simulink model "autosar_component"  (R2022b)
settings: Solver=FixedStepDiscrete  StartTime=0.0  StopTime=10.0  RelTol=1e-3
PreLoadFcn:
  | PressureEstimation = Simulink.LookupTable;
  | PressureEstimation.Table.DataType = 'auto';
  | PressureEstimation.Table.Min = -1;
  | PressureEstimation.Table.Max = 100;
  | PressureEstimation.Table.Unit = '';
  | PressureEstimation.Table.FieldName = 'Table';
  | PressureEstimation.Table.Description = ...
  |   'Pressure estimation Table data description';
  | PressureEstimation.Table.Value = ...
  |   [0.806253176323533 0.87757598601382 0.957740646602364 0.985153049483995 ...
  |    0.993888908359001 0.997089947885844 0.998445305205399 0.999091830797014 ...
  |    0.999430938454035 0.999622818995239 0.999738270814208 0.999845542107005 ...
  |    0.999937181505709 0.999967346454435 0.999979873928593 0.999985850596962 ...
  |    0.999988872471833;
  |    0.553142316928701 0.687048893636338 0.884928073705099 0.959498363205152 ...
  |    0.983356257320681 0.992081090207251 0.995771008698205 0.997530140187631 ...
  |    0.998452542678774 0.998974388477469 0.99928834538053 0.999580035742161 ...
  |    0.999829204284437 0.999911219910389 0.999945280453193 0.999961530125998 ...
  |    0.999969746130731;
  |    0.37151500208954 0.482612303368962 0.772510257347488 0.91782922063029 ...
  |    0.966202131946129 0.983928124711611 0.991420178702962 0.994990142355732 ...
  |    0.996861498829361 0.997920027607395 0.998556801019289 0.999148366829447 ...
  |    0.999653659903192 0.999819973435009 0.999889041260296 0.999921992055277 ...
  |    0.999938652267344;
  |    0.277667903102846 0.354224278507773 0.634596441906303 0.858155181125974 ...
  |    0.941196863973347 0.972020092047905 0.985064576930091 0.991280051853728 ...
  |    0.994537692220384 0.996380159664924 0.997488437655209 0.998517971150347 ...
  |    0.999397308920136 0.999686725882367 0.999806915357152 0.999864254875951 ...
  |    0.999893246159778;
  |    0.220198954206677 0.278413460665919 0.499509252438175 0.780915653069415 ...
  |    0.90725506963059 0.955734788592824 0.976359298715029 0.986196279487014 ...
  |    0.991353075497716 0.994269777477944 0.996024221776188 0.997653989166547 ...
  |    0.999045967737845 0.999504103593618 0.999694357753908 0.999785123212449 ...
  |    0.99983101483727;
  |    0.181288665766343 0.227999583948868 0.398952953853525 0.690639436957016 ...
  |    0.863705911066113 0.934478804869502 0.964951264217872 0.979525847256624 ...
  |    0.987172517967595 0.991498792106339 0.994101447273549 0.996519319760225 ...
  |    0.998584517171801 0.999264242683749 0.999546520327838 0.999681188248569 ...
  |    0.999749277343391;
  |    0.153200000488606 0.191995727776301 0.330914655151405 0.595646844312617 ...
  |    0.810666723282258 0.90775046318795 0.950492505538488 0.971050093756693 ...
  |    0.981855086965011 0.987972552524888 0.991653973147472 0.995074698970308 ...
  |    0.997996914902605 0.998958792355415 0.999358253074229 0.999548828343865 ...
  |    0.999645185116666;
  |    0.11543102087155 0.144034515174401 0.243979118856238 0.429790108547636 ...
  |    0.682438642375562 0.836880642957011 0.91118032843611 0.947813899384122 ...
  |    0.96722856464052 0.978257580098748 0.984905309066455 0.991088428442116 ...
  |    0.996374579118731 0.998115314543176 0.998838330528732 0.999183288382611 ...
  |    0.999357707498247;
  |    0.0913067476324093 0.113642314330893 0.190658230936961 0.32878428638692 ...
  |    0.545074467052933 0.74462409246358 0.856657795837454 0.91488350746312 ...
  |    0.946318097747896 0.964311517705744 0.975196237184309 0.985342971016168 ...
  |    0.994032962585561 0.996897338116608 0.998087432486324 0.998655313115969 ...
  |    0.998942465702029;
  |    0.074651918860657 0.0927600764089701 0.154689629202074 0.263508735453851 ...
  |    0.428509373032026 0.639187152983657 0.787142203938478 0.87114532382285 ...
  |    0.918076257202549 0.945327888127594 0.961925625193849 0.977463094595001 ...
  |    0.990813081836746 0.995221210749437 0.997053747988697 0.997928394076558 ...
  |    0.998370715394031;
  |    0.0625231108323717 0.0776005353603968 0.128882197432187 0.217821230748895 ...
  |    0.34926567049653 0.533026414797681 0.705799478369783 0.816462064121936 ...
  |    0.881751459546042 0.920583784269911 0.944507657720157 0.967061575702449 ...
  |    0.986544638100701 0.992996396514112 0.995680976286613 0.996962784812372 ...
  |    0.997611133655427;
  |    0.0533383634276856 0.0661461394956957 0.109538590799923 0.18412267971606 ...
  |    0.29255219843447 0.440754788055134 0.618550870186323 0.752132326009762 ...
  |    0.837127815711564 0.889546778841832 0.922421304962653 0.953755223844687 ...
  |    0.981048433857061 0.990126104885857 0.993908561852908 0.995715616100314 ...
  |    0.996629889941259;
  |    0.0461719046290558 0.057223327839534 0.0945575552493262 0.158314103258091 ...
  |    0.249955267698337 0.372825322079962 0.53225525753417 0.681013721820078 ...
  |    0.784760241136601 0.852005161999648 0.895275306545621 0.937186788001516 ...
  |    0.974139712119363 0.986508158488532 0.991672018103867 0.994141054504847 ...
  |    0.995390743685847;
  |    0.0357830207157614 0.0443099388567923 0.0730034651165902 0.121584753293742 ...
  |    0.190411497153518 0.280611299170444 0.394398141965505 0.534281588633688 ...
  |    0.663365830090947 0.758897279500008 0.825346008939808 0.893138430722029 ...
  |    0.955345741069894 0.976600929210005 0.985531654326322 0.989812926442846 ...
  |    0.991982548835214;
  |    0.0286869137234658 0.0355034233512583 0.0583848257268498 0.0969201999867393 ...
  |    0.15104654695125 0.221078862790289 0.307794324372102 0.412602365520382 ...
  |    0.536233487336572 0.649402710410808 0.736919712291059 0.833757084996449 ...
  |    0.928773563241251 0.962402265836581 0.976685081430694 0.98356210634634 ...
  |    0.987054369021;
  |    0.0235863306154347 0.0291800197474993 0.047925624770081 0.0793847279015545 ...
  |    0.123326119357344 0.179727354097858 0.248796241080163 0.331018364047279 ...
  |    0.42724438204184 0.537134400774559 0.637336655478509 0.760335336541618 ...
  |    0.893359883114823 0.943066221776258 0.964537074160009 0.97494574259801 ...
  |    0.980248325729017;
  |    0.0197778405659999 0.0244618918010893 0.0401408494783853 0.0663889743999435 ...
  |    0.1029118379984 0.149540216925307 0.206232624555673 0.273087421642731 ...
  |    0.350367228565058 0.438541144409806 0.536700025323507 0.677028641058495 ...
  |    0.848668530687683 0.917867668307508 0.948508914226248 0.96351282465758 ...
  |    0.971192248524143;
  |    0.0168486334481795 0.0208349512025066 0.0341670824865201 0.0564468168291609 ...
  |    0.0873631839769212 0.126685025043463 0.174257811754556 0.2300045810957 ...
  |    0.29393137777248 0.366138241709143 0.44683771975245 0.589975331747287 ...
  |    0.795175419924348 0.886319899213546 0.928087683613587 0.948829361164199 ...
  |    0.959515454169781];
  | PressureEstimation.BreakpointsSpecification = 'Explicit values';
  | PressureEstimation.SupportTunableSize = false;
  | PressureEstimation.Breakpoints.DataType = 'double';
  | PressureEstimation.Breakpoints.Min = [];
  | PressureEstimation.Breakpoints.Max = [];
  | PressureEstimation.Breakpoints.Unit = '';
  | PressureEstimation.Breakpoints.FieldName = 'BP1';
  | PressureEstimation.Breakpoints.Description = '';
  | PressureEstimation.Breakpoints.Value = ...
  |   [50 75 100 125 150 175 200 250 300 350 400 450 500 600 700 800 900 1000 ...
  |    ];
  | PressureEstimation.Breakpoints.TunableSizeName = 'N1';
  | PressureEstimation.Breakpoints(2).DataType = 'double';
  | PressureEstimation.Breakpoints(2).Min = [];
  | PressureEstimation.Breakpoints(2).Max = [];
  | PressureEstimation.Breakpoints(2).Unit = '';
  | PressureEstimation.Breakpoints(2).FieldName = 'BP2';
  | PressureEstimation.Breakpoints(2).Description = '';
  | PressureEstimation.Breakpoints(2).Value = ...
  |   [0 3 6 9 12 15 18 21 24 27 30 35 46 57 68 79 90];
  | PressureEstimation.Breakpoints(2).TunableSizeName = 'N2';
  | PressureEstimation.CoderInfo.StorageClass = 'Auto';
  | PressureEstimation.CoderInfo.Alias = '';
  | PressureEstimation.CoderInfo.Alignment = -1;
  | PressureEstimation.StructTypeInfo.Name = 'PressureEstimationType';
  | PressureEstimation.StructTypeInfo.DataScope = 'Auto';
  | PressureEstimation.StructTypeInfo.HeaderFileName = '';
model workspace (MATLAB code in the model file):
  | cmdLim = Simulink.Parameter;
  | cmdLim.Value = 15;
  | cmdLim.Description = 'Limit for controlling the maximum surface command angle.';
  | cmdLim.Min = 0;
  | cmdLim.Max = 90;
  | cmdLim.DocUnits = 'deg';
  | 
  | dispGain = Simulink.Parameter;
  | dispGain.Value = 0.75;
  | dispGain.Description = 'Gain applied to the displacement error.';
  | dispGain.Min = 0;
  | dispGain.Max = [];
  | dispGain.DocUnits = 'deg/sec/deg';
  | 
  | dispLim = Simulink.Parameter;
  | dispLim.Value = 30;
  | dispLim.Description = 'Limit for controlling the maximum commanded angle.';
  | dispLim.Min = 0;
  | dispLim.Max = 180;
  | dispLim.DocUnits = 'deg';
  | 
  | intGain = Simulink.Parameter;
  | intGain.Value = 0.5;
  | intGain.Description = 'Gain applied to the integral error.';
  | intGain.Min = 0;
  | intGain.Max = [];
  | intGain.DocUnits = 'deg/sec/deg/sec';
  | 
  | intLim = Simulink.Parameter;
  | intLim.Value = 5;
  | intLim.Description = 'Limit for controlling the maximum commanded angle.';
  | intLim.Min = 0;
  | intLim.Max = 90;
  | intLim.DocUnits = 'deg';
  | 
  | rateGain = Simulink.Parameter;
  | rateGain.Value = 2;
  | rateGain.Description = 'Gain applied to the rate error.';
  | rateGain.Min = 0;
  | rateGain.Max = [];
  | rateGain.DocUnits = 'deg/deg/sec';
  | 
  | rateLim = Simulink.Parameter;
  | rateLim.Value = 6;
  | rateLim.Description = 'Limit for controlling the maximum commanded angle.';
  | rateLim.Min = 0;
  | rateLim.Max = 180;
  | rateLim.DocUnits = 'deg/sec';
  | 
  | hdgGain = Simulink.Parameter;
  | hdgGain.Value = 0.015;
CloseFcn:
  | clear PressureEstimation;
settings Model: RequirementInfo={} %GIDa_fe9045fd_0412_4b6e_8206_617cc20e6fde  FPTRunName=Active  Creator=The MathWorks, Inc.  LastModifiedBy=The MathWorks, Inc.
settings SolverCC: AlgebraicLoopSolver=TrustRegion  AutoInsertRateTranBlk=on  MaxZcPerStep=1
settings DataIOCC: SaveOutput=off  SignalLogging=off  DSMLogging=off  SaveTime=off  ReturnWorkspaceOutputs=off
settings OptimizationCC: DefaultParameterBehavior=Inlined  UseDivisionForNetSlopeComputation=on  UseFloatMulNetSlope=on  UseSpecifiedMinMax=on  InlineInvariantSignals=on  EnhancedBackFolding=on  PassReuseOutputArgsAs=Individual arguments  ZeroExternalMemoryAtStartup=off  ZeroInternalMemoryAtStartup=off  NoFixptDivByZeroProtection=on  EfficientFloat2IntCast=on  OptimizeBlockOrder=speed  DifferentSizesBufferReuse=on  OptimizationCustomize=off  EfficientTunableParamExpr=on
settings DebuggingCC: ParameterTunabilityLossMsg=error  UnconnectedInputMsg=warning  UnconnectedOutputMsg=warning  UnconnectedLineMsg=warning  AllowSymbolicDim=off  SFUnexpectedBacktrackingDiag=warning  SFNoUnconditionalDefaultTransitionDiag=warning  SFExecutionAtInitializationDiag=none  SFMachineParentedDataDiag=warning  ArithmeticOperatorsInVariantConditions=warning
settings HardwareCC: ProdLongLongMode=on
settings ModelReferenceCC: EnableRefExpFcnMdlSchedulingChecks=on
settings SFSimCC: MATLABDynamicMemAlloc=off
settings RTWCC: Description=AUTOSAR  SystemTargetFile=autosar.tlc  GenCodeOnly=on  TemplateMakefile=ert_default_tmf  GenerateReport=on  RTWVerbose=off  BuildConfiguration=Faster Runs  IncludeHyperlinkInReport=on  LaunchReport=on  GenerateTraceInfo=on  GenerateTraceReport=on  GenerateTraceReportSl=on  GenerateTraceReportSf=on  GenerateTraceReportEml=on  GenerateCodeMetricsReport=on  DLArmComputeVersion=19.05
settings CodeAppCC: ForceParamTrailComments=on  IgnoreCustomStorageClasses=off  OperatorAnnotations=on  SimulinkDataObjDesc=on  SFDataObjDesc=on  CustomSymbolStrGlobalVar=rt$N$M  CustomSymbolStrType=$N$M  CustomSymbolStrFcn=$N$M$F  CustomSymbolStrMacro=$N$M  InsertBlockDesc=on  EnableCustomComments=on  ReqsInCode=on
settings STFCustomTargetCC: TargetLangStandard=C99 (ISO)  MultiwordLength=256  ParMdlRefBuildCompliant=on  CompOptLevelCompliant=on  IncludeMdlTerminateFcn=off  CombineOutputUpdateFcns=on  SuppressErrorStatus=on  ERTCustomFileBanners=on  SupportNonFinite=off  SupportComplex=off  SupportContinuousTime=off  SupportNonInlinedSFcns=off  RemoveResetFunc=on  MATLABClassNameForMDSCustomization=Simulink.SoftwareTarget.ERTCustomization  CPPClassGenCompliant=on  AutosarCompliant=on  UseToolchainInfoCompliant=on  LookupTableObjectStructAxisOrder=2,1,3,4,...  LUTObjectStructOrderEvenSpacing=Size,Table,Breakpoints  SystemTargetFile=autosar.tlc
settings ERTTargetCC: TargetLangStandard=C99 (ISO)  ConcurrentExecutionCompliant=off  IncludeMdlTerminateFcn=off  SuppressErrorStatus=on  SupportNonFinite=off  SupportComplex=off  ModelStepFunctionPrototypeControlCompliant=off  AutosarCompliant=on  LookupTableObjectStructAxisOrder=2,1,3,4,...  LUTObjectStructOrderEvenSpacing=Size,Table,Breakpoints  InlinedParameterPlacement=NonHierarchical  ERTCustomFileTemplate=example_file_process.tlc
settings ConfigComp: CovScope=ReferencedModels  CovSaveName=covdata_rollAP  CovMetricSettings=dcmtrwe  CovHTMLOptions=-sRT=1 -aTS=1 -bRG=1 -bTC=1 -hTR=1 -nFC=0 -scm=1 -bcm=1 -xEv=0  CovSaveCumulativeToWorkspaceVar=on  CovSaveSingleToWorkspaceVar=on  CovCumulativeVarName=covCumulativeData_rollAP  CovReportOnPause=off  CovExternalEMLEnable=off  CovSFcnEnable=off

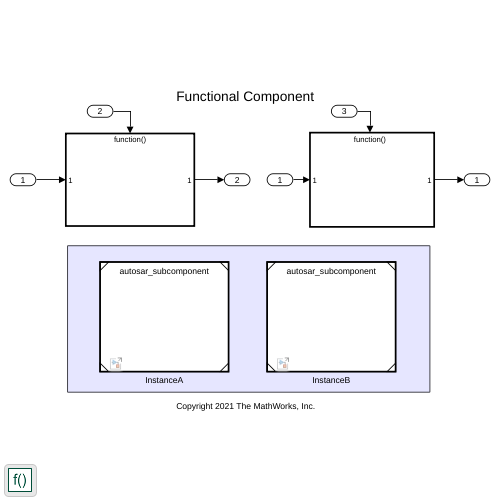
[thumbnail: Simulink's stored preview of the top-level diagram]
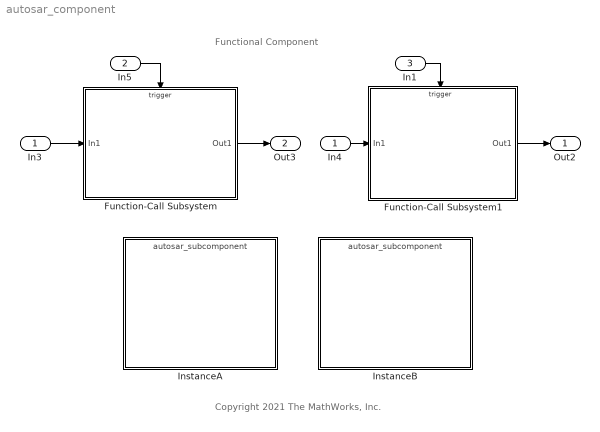
== system autosar_component ==
  note: Functional Component
  note: Copyright 2021 The MathWorks, Inc.
  In3 : Inport
  In5 : Inport  Port=2  SampleTime=0.01  OutputFunctionCall=on
  In1 : Inport  Port=3  SampleTime=0.001  OutputFunctionCall=on
  Function-Call Subsystem : Subsystem  TreatAsAtomicUnit=on
  Function-Call Subsystem1 : Subsystem  TreatAsAtomicUnit=on
  In4 : InportShadow
  InstanceA : ModelReference  ModelNameDialog=autosar_subcomponent  UsingDefaultArgumentValue=0,0,0,0  SimulationMode=Normal  ScheduleRates=on  ModelReferenceVersion=5.0
  InstanceB : ModelReference  ModelNameDialog=autosar_subcomponent  UsingDefaultArgumentValue=0,0,0,0  SimulationMode=Normal  ScheduleRates=on  ModelReferenceVersion=5.0
  Out2 : Outport  VectorParamsAs1DForOutWhenUnconnected=off
  Out3 : Outport  Port=2  VectorParamsAs1DForOutWhenUnconnected=off
  wires:
  Function-Call Subsystem1/1(Out1) -> Out2/1
  In3/1 -> Function-Call Subsystem/1(In1)
  In4/1 -> Function-Call Subsystem1/1(In1)
  In5/1 -> Function-Call Subsystem/Trigger
  In1/1 -> Function-Call Subsystem1/Trigger
  Function-Call Subsystem/1(Out1) -> Out3/1

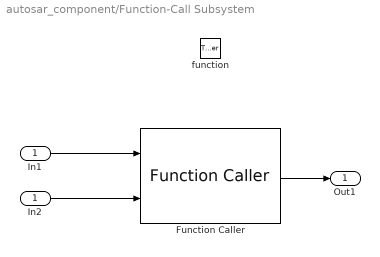
== system autosar_component/Function-Call Subsystem ==
  In1 : Inport
  function : TriggerPort  TriggerType=function-call  VariantControl=Variant
  Function Caller : FunctionCaller  FunctionPrototype=y = InstanceA.CalculateSum(u1,u2)  InputArgumentSpecifications=<Enter example>  OutputArgumentSpecifications=<Enter example>
  In2 : InportShadow
  Out1 : Outport  VectorParamsAs1DForOutWhenUnconnected=off
  wires:
  Function Caller/1 -> Out1/1
  In1/1 -> Function Caller/1
  In2/1 -> Function Caller/2

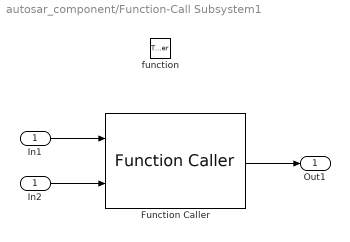
== system autosar_component/Function-Call Subsystem1 ==
  In1 : Inport
  function : TriggerPort  TriggerType=function-call  VariantControl=Variant
  Function Caller : FunctionCaller  FunctionPrototype=y = InstanceB.CalculateSum(u1,u2)  InputArgumentSpecifications=<Enter example>  OutputArgumentSpecifications=<Enter example>
  In2 : InportShadow
  Out1 : Outport  VectorParamsAs1DForOutWhenUnconnected=off
  wires:
  In1/1 -> Function Caller/1
  In2/1 -> Function Caller/2
  Function Caller/1 -> Out1/1
